simulink model "surekliModel"  (R2024a)
settings: Solver=VariableStepAuto  StartTime=0.0  StopTime=25  RelTol=1e-3
values from neighbouring files (symbols this model uses):
  b = 0.000023873    (= 2.3873e-05)    [variables.m]
  J = 0.0000023    (= 2.3e-06)    [variables.m]
  ke = 0.0000219    (= 2.19e-05)    [variables.m]
  kt = 0.0000217    (= 2.17e-05)    [variables.m]
  L = 0.000113    [variables.m]
  R = 0.199    [variables.m]
  Y1 = x7 + x6 + (x5 + x3 + x2)/(etaWG)    (= 2.3434762323e-06)    [variables.m]
  Y2 = x4/(etaWG)    (= 0.00104761904762)    [variables.m]
  Y3 = x1/(etaWG)    (= 7.68395443415e-05)    [variables.m]
libraries: slpidlib x1

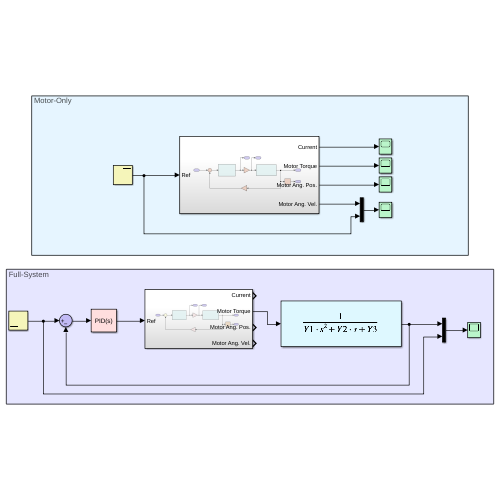
[thumbnail: Simulink's stored preview of the top-level diagram]
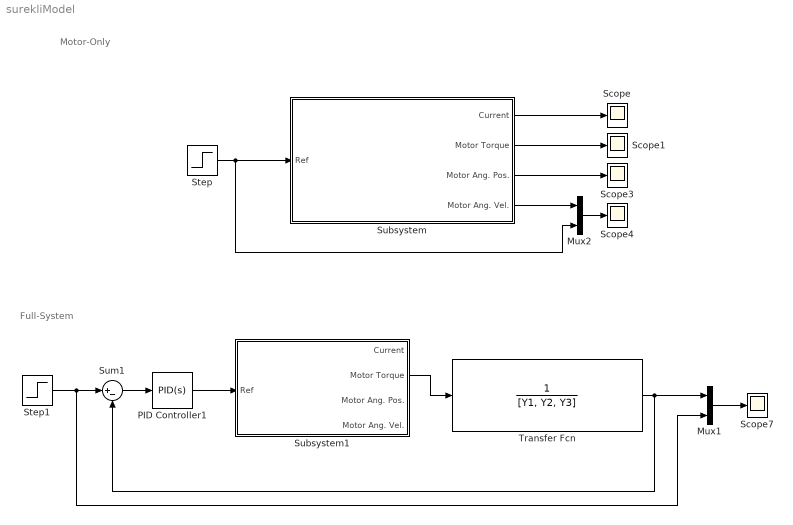
== system surekliModel ==
  note: Full-System
  note: Motor-Only
  Mux1 : Mux  Inputs=2
  Mux2 : Mux  Inputs=2
  PID Controller1 : slpidlib/PID Controller  Controller=PID  Form=Parallel  TimeDomain=Continuous-time  UseExternalTs=off  SampleTime=-1  IntegratorMethod=Forward Euler  FilterMethod=Forward Euler  ControllerParametersSource=internal  P=11.9549628360065  I=4.24350593157996  UseKiTs=off  D=-0.0810063891712427  UseExternalDerivativeSource=off  N=147.580492826738  UseFilter=on  TunerSelectOption=Transfer Function Based (PID Tuner App)  InitialConditionSource=internal  InitialConditionForIntegrator=0  InitialConditionForFilter=0  DifferentiatorICPrevScaledInput=0  ExternalReset=none  TrackingMode=off  Kt=1  LimitOutput=off  SatLimitsSource=internal  UpperSaturationLimit=inf  LowerSaturationLimit=-inf  LinearizeAsGain=on  AntiWindupMode=none  Kb=1  LimitIntegrator=off  UpperIntegratorSaturationLimit=inf  LowerIntegratorSaturationLimit=-inf  POutMin=[]  POutMax=[]  IOutMin=[]  IOutMax=[]  DOutMin=[]  DOutMax=[]  NOutMin=[]  NOutMax=[]  SumOutMin=[]  SumOutMax=[]  SaturationOutMin=[]  SaturationOutMax=[]  PParamMin=[]  PParamMax=[]  IParamMin=[]  IParamMax=[]  DParamMin=[]  DParamMax=[]  NParamMin=[]  NParamMax=[]  KbParamMin=[]  KbParamMax=[]  KtParamMin=[]  KtParamMax=[]  KbOutMin=[]  KbOutMax=[]  KtOutMin=[]  KtOutMax=[]  IntegratorOutMin=[]  IntegratorOutMax=[]  FilterOutMin=[]  FilterOutMax=[]  SumI1OutMin=[]  SumI1OutMax=[]  SumI2OutMin=[]  SumI2OutMax=[]  SumI3OutMin=[]  SumI3OutMax=[]  SumI4OutMin=[]  SumI4OutMax=[]  SumDOutMin=[]  SumDOutMax=[]  DifferentiatorOutMin=[]  DifferentiatorOutMax=[]  FilterDiffOutCoefMin=[]  FilterDiffOutCoefMax=[]  ReciprocalOutMin=[]  ReciprocalOutMax=[]  SumDenOutMin=[]  SumDenOutMax=[]  SumNumOutMin=[]  SumNumOutMax=[]  DivideOutMin=[]  DivideOutMax=[]  UdiffTsProdOutMin=[]  UdiffTsProdOutMax=[]  NTsProdOutMin=[]  NTsProdOutMax=[]  UintegralTsProdOutMin=[]  UintegralTsProdOutMax=[]  UngainTsProdOutMin=[]  UngainTsProdOutMax=[]  ClampingZeroOutDataTypeStr=Inherit: Inherit via back propagation  ClampingZeroOutMin=[]  ClampingZeroOutMax=[]  FilterDenConstantOutDataTypeStr=Inherit: Inherit via back propagation  FilterDenConstantOutMin=[]  FilterDenConstantOutMax=[]  PCopyOutDataTypeStr=Inherit: Inherit via back propagation  PCopyOutMin=[]  PCopyOutMax=[]  NCopyOutDataTypeStr=Inherit: Inherit via back propagation  NCopyOutMin=[]  NCopyOutMax=[]  IntegratorContinuousStateAttributes=''  IntegratorStateMustResolveToSignalObject=off  IntegratorRTWStateStorageClass=Auto  FilterContinuousStateAttributes=''  FilterStateMustResolveToSignalObject=off  FilterRTWStateStorageClass=Auto  ParallelPVariant=InternalParameters  IdealPVariant=Disabled  IVariant=InternalParameters  DVariant=InternalParameters  IntegratorVariant=Continuous  SatVariant=Disabled  AWVariant=Passthrough  PCopyVariant=Disabled  TRVariant=Disabled  FdbkBlocksVariant=Forward  IdealPFdbkVariant=Disabled  SatFdbkVariant=Disabled  DerivativeFilterVariant=ContFilter  NVariant=InternalParameters  NCopyVariant=Disabled  FilterICVariant=InternalICsFilter  IntegratorICVariant=InternalICs  ExternalResetVariant=Disabled  TRSumVariant=Passthrough  SumFdbkVariant=Disabled  SumVariant=Sum_PID  TsampFilterVariant=InternalTs  TsampNgainVariant=Passthrough  TsampIntegralVariant=Disabled_SignalSpec  ExternalSaturationOutDataTypeStr=Inherit: Same as second input  DerivativeSourceVariant=ErrorSignal
  Scope{,1,3..4,7} (5 alike) : Scope
  Step : Step  SampleTime=0
  Step1 : Step  After=10  SampleTime=0
  Subsystem : Subsystem
  Subsystem1 : Subsystem
  Sum1 : Sum  Inputs=|+-
  Transfer Fcn : TransferFcn  Denominator=[Y1, Y2, Y3]
  wires:
  Subsystem/1(Current) -> Scope/1
  Subsystem/2(Motor Torque) -> Scope1/1
  Subsystem/3(Motor Ang. Pos.) -> Scope3/1
  Subsystem/4(Motor Ang. Vel.) -> Mux2/1
  Sum1/1 -> PID Controller1/1
  Step1/1 -> Mux1/2, Sum1/1
  Step/1 -> Subsystem/1(Ref), Mux2/2
  Mux2/1 -> Scope4/1
  PID Controller1/1 -> Subsystem1/1(Ref)
  Transfer Fcn/1 -> Mux1/1, Sum1/2
  Mux1/1 -> Scope7/1
  Subsystem1/2(Motor Torque) -> Transfer Fcn/1

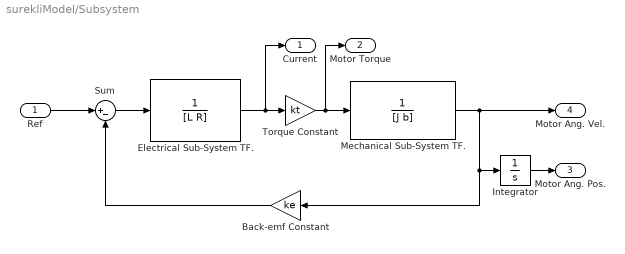
== system surekliModel/Subsystem ==
  Ref : Inport
  "Back-emf Constant " : Gain  Gain=ke
  Electrical Sub-System TF. : TransferFcn  Denominator=[L R]
  Integrator : Integrator
  Mechanical Sub-System TF. : TransferFcn  Denominator=[J b]
  Sum : Sum  Inputs=|+-
  Torque Constant : Gain  Gain=kt
  Current : Outport
  Motor Torque : Outport  Port=2
  Motor Ang. Pos. : Outport  Port=3
  Motor Ang. Vel. : Outport  Port=4
  wires:
  Torque Constant/1 -> Motor Torque/1, Mechanical Sub-System TF./1
  Sum/1 -> Electrical Sub-System TF./1
  "Back-emf Constant "/1 -> Sum/2
  Ref/1 -> Sum/1
  Electrical Sub-System TF./1 -> Current/1, Torque Constant/1
  Integrator/1 -> Motor Ang. Pos./1
  Mechanical Sub-System TF./1 -> Integrator/1, "Back-emf Constant "/1, Motor Ang. Vel./1

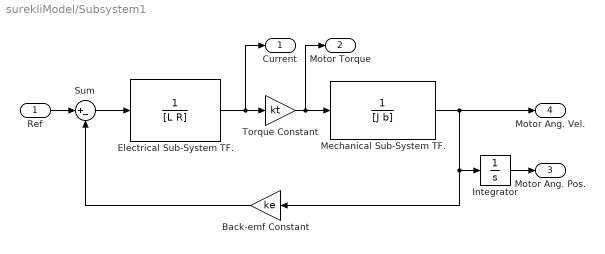
== system surekliModel/Subsystem1 ==
  Ref : Inport
  "Back-emf Constant " : Gain  Gain=ke
  Electrical Sub-System TF. : TransferFcn  Denominator=[L R]
  Integrator : Integrator
  Mechanical Sub-System TF. : TransferFcn  Denominator=[J b]
  Sum : Sum  Inputs=|+-
  Torque Constant : Gain  Gain=kt
  Current : Outport
  Motor Torque : Outport  Port=2
  Motor Ang. Pos. : Outport  Port=3
  Motor Ang. Vel. : Outport  Port=4
  wires:
  Torque Constant/1 -> Motor Torque/1, Mechanical Sub-System TF./1
  Sum/1 -> Electrical Sub-System TF./1
  "Back-emf Constant "/1 -> Sum/2
  Ref/1 -> Sum/1
  Electrical Sub-System TF./1 -> Current/1, Torque Constant/1
  Integrator/1 -> Motor Ang. Pos./1
  Mechanical Sub-System TF./1 -> Integrator/1, "Back-emf Constant "/1, Motor Ang. Vel./1
